simulink model "mod_sl_quadrotor_V2"  (R2017b)
settings: Solver=ode45  StartTime=0.0  StopTime=5  MaxStep=0.1  RelTol=1e-3  EnableMultiTasking=on
PreLoadFcn:
  | % load parameters of the default quadrotor
  | disp('Quadrotor parameters loaded by PreLoadFcn')
  | mdl_quadrotor
undefined symbols (not defined in the file): psi, quadrotor, rot2, x, y, z
libraries: NLGCToolbox x6, roblocks x2, simulink x2
settings Model: Creator=corkep  LastModifiedBy=hoang
settings DataIOCC: LimitDataPoints=on
settings OptimizationCC: ExpressionDepthLimit=2147483647  LifeSpan=inf
settings DebuggingCC: UnderspecifiedInitializationDetection=Classic  MergeDetectMultiDrivingBlocksExec=none  SolverPrmCheckMsg=warning  AllowSymbolicDim=off  StateNameClashWarn=warning  SFUnexpectedBacktrackingDiag=warning  SFNoUnconditionalDefaultTransitionDiag=warning  SFExecutionAtInitializationDiag=none
settings HardwareCC: ProdBitPerPointer=32  ProdBitPerSizeT=32  ProdBitPerPtrDiffT=32  ProdLargestAtomicFloat=None  ProdIntDivRoundTo=Undefined  ProdEndianess=Unspecified  ProdWordSize=32  ProdHWDeviceType=32-bit Generic
settings ModelReferenceCC: PropagateSignalLabelsOutOfModel=off
settings CodeAppCC: StateflowObjectComments=on
settings GRTTargetCC: TargetLangStandard=C89/C90 (ANSI)  GeneratePreprocessorConditionals=Disable all  CombineOutputUpdateFcns=off  GRTInterface=on
settings ConfigComp: CovMetricSettings=dw  CovHtmlReporting=on  CovSaveCumulativeToWorkspaceVar=on  CovSaveSingleToWorkspaceVar=on  CovExternalEMLEnable=off  CovSFcnEnable=off

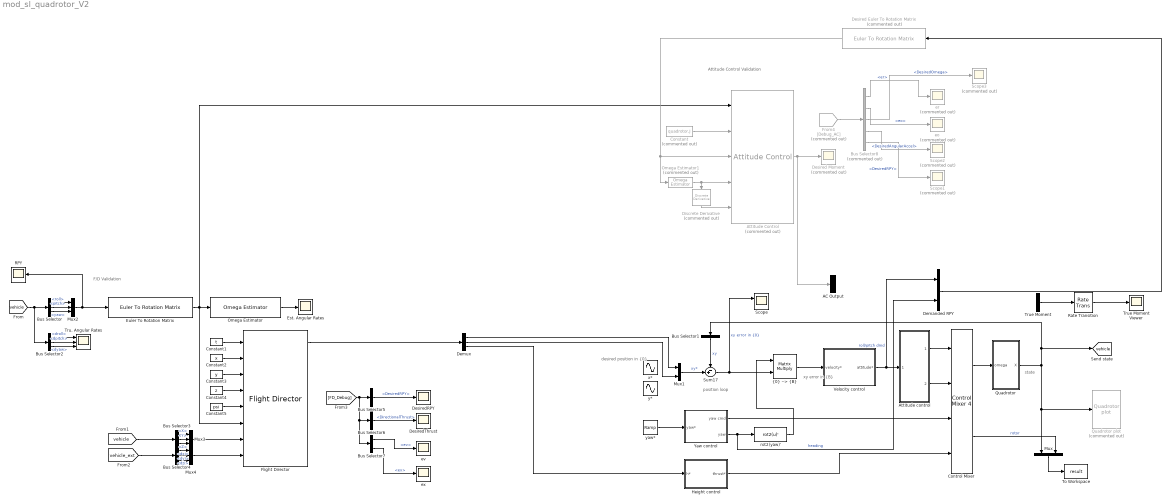
== system mod_sl_quadrotor_V2 ==
  note: Attitude Control Validation
  note: F/D Validation
  note: xy error
      | in {B}
  note: desired position
      | in {0}
  note: position
      | loop
  note: state
  AC Output : Demux  Outputs=3
  Attitude Control : NLGCToolbox/Attitude Control  Commented=on  kr=64  ko=1.25  Ts=1/120
      settings: SourceProductName=Thinh - NLGC for Quadrotor
  Attitude control : Subsystem  mask{P=100, D=1}
      mask prompts: P "Proportional gain"; D "Derivative gain"
  Bus Selector : BusSelector  OutputSignals=roll,pitch,yaw
  Bus Selector1 : BusSelector  OutputSignals=X,Y  OutputAsBus=on
  Bus Selector2 : BusSelector  OutputSignals=droll,dpitch,dyaw
  Bus Selector3 : BusSelector  OutputSignals=X,Y,Z
  Bus Selector4 : BusSelector  OutputSignals=dxi,dyi,dzi
  Bus Selector5 : BusSelector  OutputSignals=DesiredRPY
  Bus Selector6 : BusSelector  OutputSignals=DirectionalThrust
  Bus Selector7 : BusSelector  OutputSignals=ev,ex
  Bus Selector8 : BusSelector  Commented=on  OutputSignals=er,eo,DesiredOmega,DesiredAngularAccel,DesiredRPY
  Constant : Constant  Commented=on  Value=quadrotor.J
  Constant1 : Constant  Value=t
  Constant2 : Constant  Value=x
  Constant3 : Constant  Value=y
  Constant4 : Constant  Value=z
  Constant5 : Constant  Value=psi
  Control Mixer : roblocks/Vehicles/Control Mixer 4  quad=quadrotor  maxrot=1000  minrot=5
  Demanded RPY : Mux  Inputs=2
  Demux : Demux  Outputs=3
  Desired Euler To Rotation Matrix : NLGCToolbox/Euler To Rotation Matrix  Commented=on
      settings: SourceProductName=Thinh - NLGC for Quadrotor
  Desired Moment : Scope  Commented=on
  DesiredRPY : Scope
  DesiredThrust : Scope
  Discrete Derivative : simulink/Discrete/Discrete Derivative  Commented=on  gainval=1  ICPrevScaledInput=0.0  OutMin=[]  OutMax=[]  OutDataType=fixdt(1, 16)  OutScaling=2^-10  DoSatur=off
  Est. Angular Rates : Scope
  Euler To Rotation Matrix : NLGCToolbox/Euler To Rotation Matrix
      settings: SourceProductName=Thinh - NLGC for Quadrotor
  Flight Director : NLGCToolbox/Flight Director  Ts=1/120  kx=16.4  kv=3.8
      settings: SourceProductName=Thinh - NLGC for Quadrotor
  From4 : From  Commented=on  GotoTag=Debug_AC  TagVisibility=global
  Height control : Subsystem  mask{P=4, D=1, T0=40}
      mask prompts: P "Proportional gain"; D "Derivative gain"; T0 "Thrust feedforward"
  Mux : Mux  Inputs=2
  Mux1 : Mux  Inputs=2
  Mux2 : Mux  Inputs=3
  Mux3 : Mux  Inputs=3
  Mux4 : Mux  Inputs=3
  Omega Estimator : NLGCToolbox/Omega Estimator  Ts=1/120
      settings: SourceProductName=Thinh - NLGC for Quadrotor
  Omega Estimator1 : NLGCToolbox/Omega Estimator  Commented=on  Ts=1/120
      settings: SourceProductName=Thinh - NLGC for Quadrotor
  Quadrotor : Subsystem  AncestorBlock=roblocks/Vehicles/Quadrotor  mask{quad=quadrotor, x0=[0 0 -4], groundflag=on}
      mask prompts: quad "Quadrotor params"; x0 "Initial position"; groundflag "Ground"
      mask help: Quadrotor dynamics
      mask Help:
      | Integrate spatial velocity to update pose represented as a homogeneous
      | transformation.
      | 
      | <b>Parameters::</b>
      | 
      | q (struct)  A structure containing quadrotor dynamics
      | 
      | The elements of q are:
      | 
      |  J         Flyer rotational inertia matrix (3x3)
      |  h         Height of rotors above CoG (1x1)
      |  d         Length of flyer arms (1x1)
      |  nb        Number of blades per rotor (1x1)
      |  r         Rotor radius (1x1)
      |  c         Blade chord (1x1)
      |  e         Flapping hinge offset (1x1)
      |  Mb        Rotor blade mass (1x1)
      |  Mc        Estimated hub clamp mass (1x1)
      |  ec        Blade root clamp displacement (1x1)
      |  Ib        Rotor blade rotational inertia (1x1)
      |  Ic        Estimated root clamp inertia (1x1)
      |  mb        Static blade moment (1x1)
      |  Ir        Total rotor inertia (1x1)
      |  Ct        Non-dim. thrust coefficient (1x1)
      |  Cq        Non-dim. torque coefficient (1x1)
      |  sigma     Rotor solidity ratio (1x1)
      |  thetat    Blade tip angle (1x1)
      |  theta0    Blade root angle (1x1)
      |  theta1    Blade twist angle (1x1)
      |  theta75   3/4 blade angle (1x1)
      |  thetai    Blade ideal root approximation (1x1)
      |  a         Lift slope gradient (1x1)
      |  A         Rotor disc area (1x1)
      |  gamma     Lock number (1x1)
      | 
      | 
      | <b>Inputs::</b>
      | 
      | w1 (1x1) angular velocity of rotor 1 [rad]
      | w2 (1x1) angular velocity of rotor 2 [rad]
      | w3 (1x1) angular velocity of rotor 3 [rad]
      | w4 (1x1) angular velocity of rotor 4 [rad]
      | 
      | <b>Outputs::</b>
      | 
      | X (1x12) state vector (x, y, z, thr, thp, thy, xd, yd, zd, thrd, thpd, thyd)
      | 
      | (x,y,z) is the position in the world frame [m]
      | (thr, thp, thy) the roll/pitch/yaw orientation in the world frame [rad]
      | (xd,yd,zd) is the velocity in the body frame [m]
      | (thrd,thpd,thyd) is the roll/pitch/yaw rates in the body frame [rad/s]
      | 
      | <b>Notes::</b>
      | 
      | - See also mdl_quadrotor which defines parameters for the ANU X4 flyer.
      mask Display:
      | port_label('input',1,'\varpi','texmode','on');
      | port_label('output',1,'X','texmode','on');
  Quadrotor plot : roblocks/Vehicles/Quadrotor plot  Commented=on  quad=quadrotor  xydim=2  zdim=10
  RPY : Scope
  Rate Transition : RateTransition  OutPortSampleTime=1/120
  Scope : Scope  NumInputPorts=2
  Scope1 : Scope  Commented=on
  Scope2 : Scope  Commented=on
  Scope3 : Scope  Commented=on
  Sum17 : Sum  Inputs=-+|
  To Workspace : ToWorkspace  VariableName=result  SampleTime=-1
  Tru. Angular Rates : Scope  NumInputPorts=3
  True Moment : Mux  Inputs=3
  True Moment Viewer : Scope
  Velocity control : Subsystem  mask{P=0.1, D=2}
      mask prompts: P "Proportional gain"; D "Derivative gain"
  Yaw control : Subsystem  mask{P=20, D=2}
      mask prompts: P "Proportional gain"; D "Derivative gain"
  eo : Scope  Commented=on
  er : Scope  Commented=on
  ev : Scope
  ex : Scope
  rot2(yaw)' : MATLABFcn  MATLABFcn=rot2(u)'  OutputDimensions=[2 2]  Output1D=off
  x* : Sin  Frequency=2*pi*.125  Phase=-pi/2  SampleTime=0
  y* : Sin  Amplitude=0  Frequency=2*pi*.125  SampleTime=0
  yaw* : simulink/Sources/Ramp  slope=0.5  start=2  X0=0
  "{0} --> {B}" : Product  Multiplication=Matrix(*)  RndMeth=Zero
  tag scope: vehicle=global
  wires:
  Quadrotor/1(X) -> Quadrotor plot/1, Mux/1, [vehicle], Bus Selector1/1
  Mux/1 -> To Workspace/1
  Control Mixer/2 -> Mux/2  "rotor"
  Sum17/1 -> Scope/1, "{0} --> {B}"/2  "xy error in {0}"
  "{0} --> {B}"/1 -> Velocity control/1(velocity*)
  Velocity control/1(attitude*) -> Demanded RPY/1, Attitude control/1(attitude*)  "roll/pitch dmd"
  Yaw control/2(yaw) -> Demanded RPY/2, rot2(yaw)'/1  "heading"
  yaw*/1 -> Yaw control/1(yaw*)
  Mux1/1 -> Sum17/2  "xy*"
  Bus Selector1/1 -> Sum17/1  "xy"
  rot2(yaw)'/1 -> "{0} --> {B}"/1
  Control Mixer/1 -> Quadrotor/1(omega)
  Height control/1(thrust*) -> Control Mixer/4
  Euler To Rotation Matrix/1 -> Attitude Control/1, Flight Director/6, Omega Estimator/1
  Bus Selector/1 -> Mux2/1  "<roll>"
  Bus Selector/2 -> Mux2/2  "<pitch>"
  Bus Selector/3 -> Mux2/3  "<yaw>"
  Mux2/1 -> RPY/1, Euler To Rotation Matrix/1
  Omega Estimator/1 -> Est. Angular Rates/1
  [vehicle] -> Bus Selector2/1, Bus Selector/1
  Bus Selector2/1 -> Tru. Angular Rates/1  "<droll>"
  Bus Selector2/2 -> Tru. Angular Rates/2  "<dpitch>"
  Bus Selector2/3 -> Tru. Angular Rates/3  "<dyaw>"
  Constant1/1 -> Flight Director/1
  Constant2/1 -> Flight Director/2
  Constant3/1 -> Flight Director/3
  Constant4/1 -> Flight Director/4
  Constant5/1 -> Flight Director/5
  [vehicle] -> Bus Selector3/1
  Bus Selector3/1 -> Mux3/1  "<X>"
  Bus Selector3/2 -> Mux3/2  "<Y>"
  Bus Selector3/3 -> Mux3/3  "<Z>"
  Mux3/1 -> Flight Director/7
  [vehicle_ext] -> Bus Selector4/1
  Bus Selector4/1 -> Mux4/1  "<dxi>"
  Bus Selector4/2 -> Mux4/2  "<dyi>"
  Bus Selector4/3 -> Mux4/3  "<dzi>"
  Mux4/1 -> Flight Director/8
  [FD_Debug] -> Bus Selector7/1, Bus Selector6/1, Bus Selector5/1
  Bus Selector5/1 -> DesiredRPY/1  "<DesiredRPY>"
  Bus Selector6/1 -> DesiredThrust/1  "<DirectionalThrust>"
  Bus Selector7/1 -> ev/1  "<ev>"
  Bus Selector7/2 -> ex/1  "<ex>"
  Flight Director/1 -> Demux/1
  Demux/1 -> Mux1/1
  Demux/2 -> Mux1/2
  Demux/3 -> Height control/1(h*)
  Constant/1 -> Attitude Control/2
  Desired Euler To Rotation Matrix/1 -> Attitude Control/3, Omega Estimator1/1
  Demanded RPY/1 -> Desired Euler To Rotation Matrix/1
  Omega Estimator1/1 -> Discrete Derivative/1, Attitude Control/4
  Discrete Derivative/1 -> Attitude Control/5
  Attitude Control/1 -> Desired Moment/1, AC Output/1
  True Moment/1 -> Rate Transition/1
  Rate Transition/1 -> True Moment Viewer/1
  From4/1 -> Bus Selector8/1
  Bus Selector8/5 -> Scope1/1  "<DesiredRPY>"
  Bus Selector8/4 -> Scope2/1  "<DesiredAngularAccel>"
  Bus Selector8/3 -> Scope3/1  "<DesiredOmega>"
  Bus Selector8/1 -> er/1  "<er>"
  Bus Selector8/2 -> eo/1  "<eo>"
  Attitude control/1(roll torque*) -> Control Mixer/1
  Attitude control/2(pitch torque*) -> Control Mixer/2
  Yaw control/1(yaw cmd) -> Control Mixer/3

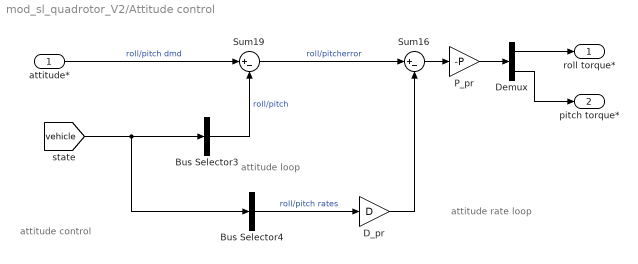
== system mod_sl_quadrotor_V2/Attitude control ==
  note: attitude control
  note: attitude rate loop
  note: attitude loop
  attitude* : Inport
  Bus Selector3 : BusSelector  OutputSignals=roll,pitch  OutputAsBus=on
  Bus Selector4 : BusSelector  OutputSignals=droll,dpitch  OutputAsBus=on
  D_pr : Gain  Gain=D
  Demux : Demux  Outputs=2
  P_pr : Gain  Gain=-P
  Sum16 : Sum  Inputs=|+-
  Sum19 : Sum  Inputs=|+-
  roll torque* : Outport
  pitch torque* : Outport  Port=2
  wires:
  [vehicle] -> Bus Selector4/1, Bus Selector3/1
  attitude*/1 -> Sum19/1  "roll/pitch dmd"
  Bus Selector3/1 -> Sum19/2  "roll/pitch"
  Bus Selector4/1 -> D_pr/1  "roll/pitch rates"
  Sum19/1 -> Sum16/1  "roll/pitcherror"
  Sum16/1 -> P_pr/1
  P_pr/1 -> Demux/1
  D_pr/1 -> Sum16/2
  Demux/2 -> pitch torque*/1
  Demux/1 -> roll torque*/1

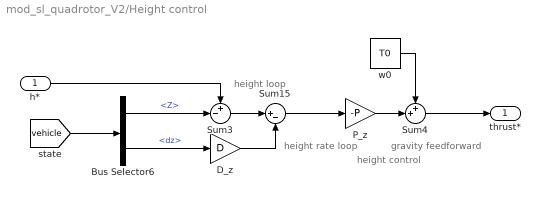
== system mod_sl_quadrotor_V2/Height control ==
  note: height control
  note: gravity feedforward
  note: height rate
      | loop
  note: height
      | loop
  h* : Inport
  Bus Selector6 : BusSelector  OutputSignals=Z,dz
  D_z : Gain  Gain=D
  P_z : Gain  Gain=-P
  Sum15 : Sum  Inputs=|+-
  Sum3 : Sum  Inputs=+-|
  Sum4 : Sum  Inputs=++|
  w0 : Constant  Value=T0  SampleTime=0
  thrust* : Outport
  wires:
  w0/1 -> Sum4/1
  Sum15/1 -> P_z/1
  P_z/1 -> Sum4/2
  Bus Selector6/1 -> Sum3/2  "<Z>"
  h*/1 -> Sum3/1
  Sum3/1 -> Sum15/1
  Bus Selector6/2 -> D_z/1  "<dz>"
  D_z/1 -> Sum15/2
  Sum4/1 -> thrust*/1
  [vehicle] -> Bus Selector6/1

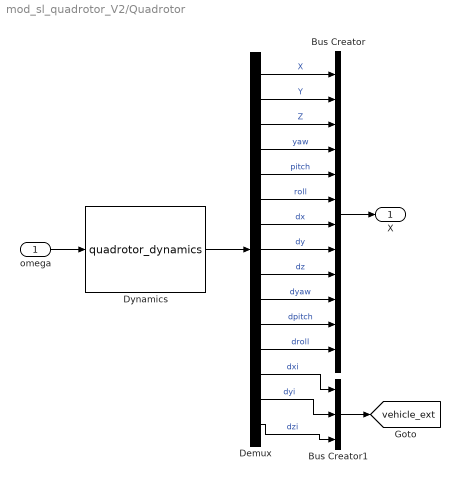
== system mod_sl_quadrotor_V2/Quadrotor ==
  omega : Inport
  Bus Creator : BusCreator  Inputs='X','Y','Z','yaw','pitch','roll','dx','dy','dz','dyaw','dpitch','droll'
  Bus Creator1 : BusCreator  Inputs=3
  Demux : Demux  Outputs=15
  Dynamics : S-Function  FunctionName=quadrotor_dynamics  Parameters=quad, x0, groundflag  SFunctionDeploymentMode=off  EnableBusSupport=off
  X : Outport
  tag scope: vehicle_ext=global
  wires:
  Demux/1 -> Bus Creator/1  "X"
  Demux/3 -> Bus Creator/3  "Z"
  Demux/4 -> Bus Creator/4  "yaw"
  Demux/5 -> Bus Creator/5  "pitch"
  omega/1 -> Dynamics/1
  Demux/7 -> Bus Creator/7  "dx"
  Demux/9 -> Bus Creator/9  "dz"
  Demux/2 -> Bus Creator/2  "Y"
  Demux/6 -> Bus Creator/6  "roll"
  Demux/8 -> Bus Creator/8  "dy"
  Bus Creator/1 -> X/1
  Dynamics/1 -> Demux/1
  Demux/10 -> Bus Creator/10  "dyaw"
  Demux/11 -> Bus Creator/11  "dpitch"
  Demux/12 -> Bus Creator/12  "droll"
  Demux/13 -> Bus Creator1/1  "dxi"
  Demux/14 -> Bus Creator1/2  "dyi"
  Demux/15 -> Bus Creator1/3  "dzi"
  Bus Creator1/1 -> [vehicle_ext]

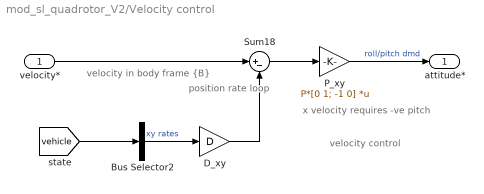
== system mod_sl_quadrotor_V2/Velocity control ==
  note: x velocity requires -ve pitch
  note: velocity in body frame {B}
  note: velocity control
  note: position rate
      | loop
  velocity* : Inport
  Bus Selector2 : BusSelector  OutputSignals=dx,dy  OutputAsBus=on
  D_xy : Gain  Gain=D
  P_xy : Gain  Gain=P*[0 1; -1 0]  Multiplication=Matrix(K*u)
  Sum18 : Sum  Inputs=|+-
  attitude* : Outport
  wires:
  Bus Selector2/1 -> D_xy/1  "xy rates"
  D_xy/1 -> Sum18/2
  Sum18/1 -> P_xy/1
  velocity*/1 -> Sum18/1
  [vehicle] -> Bus Selector2/1
  P_xy/1 -> attitude*/1  "roll/pitch dmd"

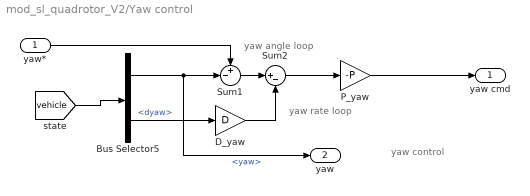
== system mod_sl_quadrotor_V2/Yaw control ==
  note: yaw control
  note: yaw rate
      | loop
  note: yaw angle
      | loop
  yaw* : Inport
  Bus Selector5 : BusSelector  OutputSignals=yaw,dyaw
  D_yaw : Gain  Gain=D
  P_yaw : Gain  Gain=-P
  Sum1 : Sum  Inputs=+-|
  Sum2 : Sum  Inputs=|+-
  yaw cmd : Outport
  yaw : Outport  Port=2
  wires:
  [vehicle] -> Bus Selector5/1
  P_yaw/1 -> yaw cmd/1
  Bus Selector5/1 -> yaw/1, Sum1/2  "<yaw>"
  Sum2/1 -> P_yaw/1
  Bus Selector5/2 -> D_yaw/1  "<dyaw>"
  D_yaw/1 -> Sum2/2
  Sum1/1 -> Sum2/1
  yaw*/1 -> Sum1/1
